simulink library "lib_Differential"  (R2017a)
settings: Solver=VariableStepAuto  StartTime=0.0  StopTime=10.0  RelTol=1e-3
undefined symbols (not defined in the file): fd, GearBox
settings Model: Creator=Di Russo  LastModifiedBy=Vraj M

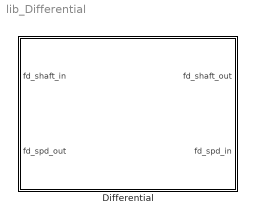
== system lib_Differential ==
  Differential : Subsystem
      mask Display:
      | image('Images/Diff.jpg');
      | color('red');
      | port_label('input',1,'ShaftIn')
      | port_label('input',2,'SpdOut')
      | port_label('output',1,'ShaftOut')
      | port_label('output',2,'SpdIn')

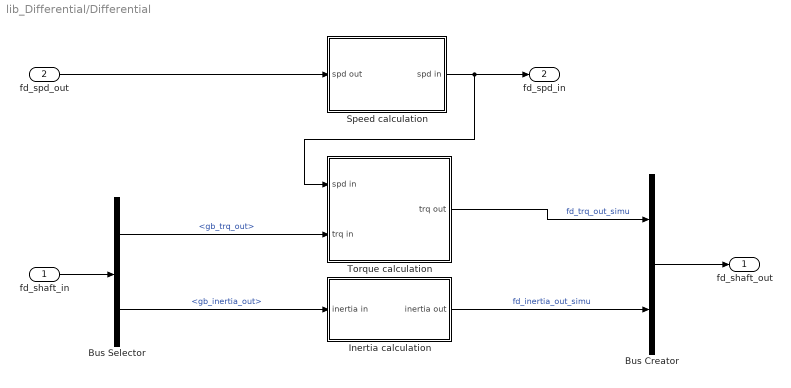
== system lib_Differential/Differential ==
  fd_shaft_in : Inport
  fd_spd_out : Inport  Port=2
  Bus Creator : BusCreator  Inputs=2
  Bus Selector : BusSelector  OutputSignals=gb_trq_out,gb_inertia_out
  Inertia calculation : Subsystem
  Speed calculation : Subsystem
  Torque calculation : Subsystem
  fd_shaft_out : Outport
  fd_spd_in : Outport  Port=2
  wires:
  Bus Creator/1 -> fd_shaft_out/1
  fd_shaft_in/1 -> Bus Selector/1
  Bus Selector/2 -> Inertia calculation/1(inertia in)  "<gb_inertia_out>"
  Bus Selector/1 -> Torque calculation/2(trq in)  "<gb_trq_out>"
  Inertia calculation/1(inertia out) -> Bus Creator/2  "fd_inertia_out_simu"
  Speed calculation/1(spd in) -> fd_spd_in/1, Torque calculation/1(spd in)
  fd_spd_out/1 -> Speed calculation/1(spd out)
  Torque calculation/1(trq out) -> Bus Creator/1  "fd_trq_out_simu"

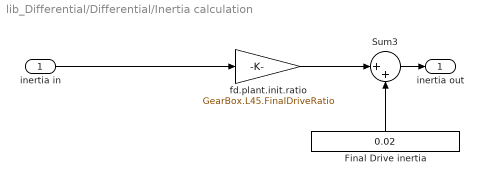
== system lib_Differential/Differential/Inertia calculation ==
  inertia in : Inport
  Final Drive inertia : Constant  Value=0.02
  Sum3 : Sum  Inputs=|++  SaturateOnIntegerOverflow=on  InputSameDT=on  OutDataTypeStr=Inherit: Same as first input
  "fd.plant.init.ratio " : Gain  Gain=GearBox.L45.FinalDriveRatio  SaturateOnIntegerOverflow=on  OutDataTypeStr=Inherit: Same as input  ParamDataTypeStr=Inherit: Same as input
  inertia out : Outport
  wires:
  inertia in/1 -> "fd.plant.init.ratio "/1
  Sum3/1 -> inertia out/1
  Final Drive inertia/1 -> Sum3/2
  "fd.plant.init.ratio "/1 -> Sum3/1

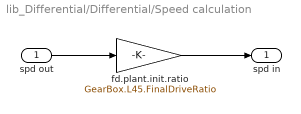
== system lib_Differential/Differential/Speed calculation ==
  spd out : Inport
  fd.plant.init.ratio : Gain  Gain=GearBox.L45.FinalDriveRatio  SaturateOnIntegerOverflow=on  OutDataTypeStr=Inherit: Same as input  ParamDataTypeStr=Inherit: Same as input
  spd in : Outport
  wires:
  fd.plant.init.ratio/1 -> spd in/1
  spd out/1 -> fd.plant.init.ratio/1

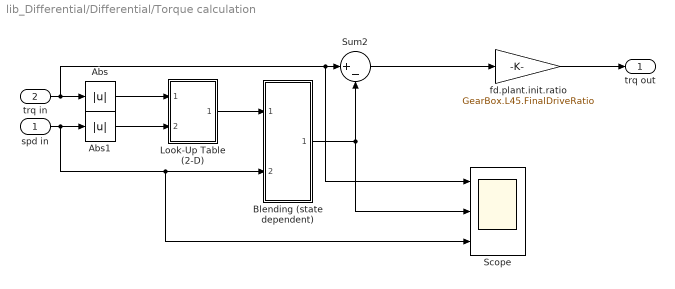
== system lib_Differential/Differential/Torque calculation ==
  spd in : Inport
  trq in : Inport  Port=2
  Abs : Abs  SaturateOnIntegerOverflow=on
  Abs1 : Abs  SaturateOnIntegerOverflow=on
  Blending (state dependent) : Subsystem  mask(State dependent blending){xl=-fd.plant.init.spd_thresh, yl=-1, xc=0, yc=0, xr=fd.plant.init.spd_thresh, yr=1}
      mask prompts: xl "Left point (x):"; yl "Left point (y):"; xc "Center point (x):"; yc "Center point (y):"; xr "Right point (x):"; yr "Right point (y):"
      mask help: This block implements state dependent smoothing/blending. IMPORTANT: See help menu.
      mask Help: The output equals the product of the first input and a "hat" function defined by the three points specified in the dialog box.  The second input forms the argument to the hat function.\n\nIMPORTANT: A divide by zero error will result if first coordinates of the three points specified for the hat function are NOT distinct.
      mask Display: plot([-1 1 3 6 8], [1.5 1.5 0.5 4.0 4.0])
  Look-Up Table (2-D) : Subsystem  mask(Lookup Table (2-D)){x=fd.plant.init.trq_loss.idx1_trq, y=fd.plant.init.trq_loss.idx2_spd, t=fd.plant.init.trq_loss.map}
      mask prompts: x "Row:"; y "Column:"; t "Table:"
      mask help: Performs 2-D linear interpolation of input values using the specified input/output table. Extrapolation is performed outside the table boundaries.
      mask init:
      | [r,c]=size(t);
      | xt=reshape(x,prod(size(x)),1);
      | xi=xt(:,ones(1,c));
      | minx=min(x); maxx=max(x);
      | mint=min(min(t)); maxt=max(max(t));
      mask Display: plot(xi,t,[minx maxx],[mint mint],[minx minx],[mint maxt])
  Scope : Scope  NumInputPorts=3
  Sum2 : Sum  Inputs=|+-  SaturateOnIntegerOverflow=on  InputSameDT=on  OutDataTypeStr=Inherit: Same as first input
  fd.plant.init.ratio : Gain  Gain=GearBox.L45.FinalDriveRatio  SaturateOnIntegerOverflow=on  OutDataTypeStr=Inherit: Same as input  ParamDataTypeStr=Inherit: Same as input
  trq out : Outport
  wires:
  spd in/1 -> Blending (state dependent)/2(Control (state)), Scope/3, Abs1/1
  fd.plant.init.ratio/1 -> trq out/1
  Sum2/1 -> fd.plant.init.ratio/1
  trq in/1 -> Sum2/1, Scope/1, Abs/1
  Blending (state dependent)/1(Output) -> Scope/2, Sum2/2
  Look-Up Table (2-D)/1(Out1) -> Blending (state dependent)/1(Input)
  Abs1/1 -> Look-Up Table (2-D)/2(Cols)
  Abs/1 -> Look-Up Table (2-D)/1(Rows)

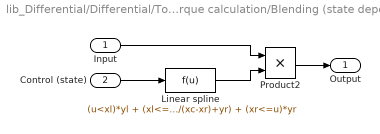
== system lib_Differential/Differential/Torque calculation/Blending (state dependent) ==
  Input : Inport
  Control (state) : Inport  Port=2
  Linear spline : Fcn  Expr=(u<xl)*yl + (xl<=u)*(u<xc)*((yc-yl)*(u-xl)/(xc-xl)+yl) + (xc<=u)*(u<xr)*((yc-yr)*(u-xr)/(xc-xr)+yr) + (xr<=u)*yr
  Product2 : Product  SaturateOnIntegerOverflow=on  InputSameDT=on  OutDataTypeStr=Inherit: Same as first input
  Output : Outport
  wires:
  Control (state)/1 -> Linear spline/1
  Product2/1 -> Output/1
  Linear spline/1 -> Product2/2
  Input/1 -> Product2/1

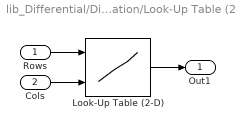
== system lib_Differential/Differential/Torque calculation/Look-Up Table (2-D) ==
  Rows : Inport
  Cols : Inport  Port=2
  Look-Up Table (2-D) : Lookup2D  RowIndex=x  ColumnIndex=y  Table=t  SaturateOnIntegerOverflow=on  InputSameDT=on
  Out1 : Outport
  wires:
  Look-Up Table (2-D)/1 -> Out1/1
  Cols/1 -> Look-Up Table (2-D)/2
  Rows/1 -> Look-Up Table (2-D)/1
